simulink subsystem "Sensores_IR"  (R2023b)
settings: Solver=VariableStepAuto  StartTime=0.0  StopTime=10.0  RelTol=1e-3
libraries: arduinolib x2
settings Model: Creator=Usuario_UMA  LastModifiedBy=javie

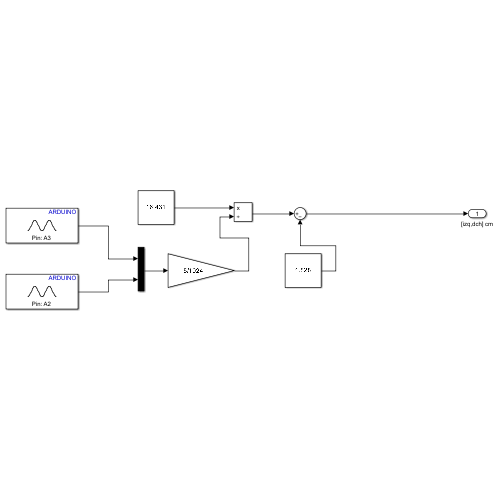
[thumbnail: Simulink's stored preview of the top-level diagram]
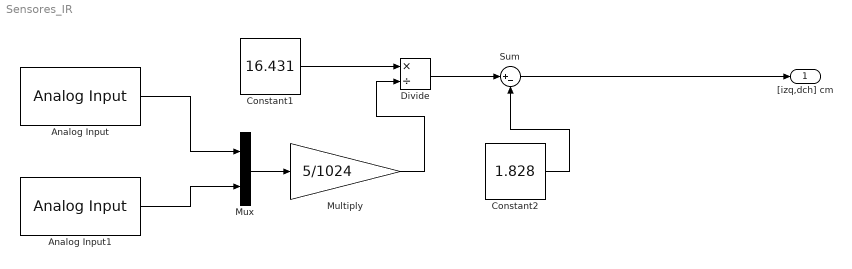
== system Sensores_IR ==
  Analog Input : arduinolib/Analog Input  pinNumber=3  ReadResultsOnly=off  ConversionTriggerSource=Software  ExternalTriggerType=uint32( 0 )  OutputDataType=uint16  EnableConversionCompleteNotify=off  EnableOuputStatus=off  SampleTime=-1  blockPlatform=arduino
  Analog Input1 : arduinolib/Analog Input  pinNumber=2  ReadResultsOnly=off  ConversionTriggerSource=Software  ExternalTriggerType=uint32( 0 )  OutputDataType=uint16  EnableConversionCompleteNotify=off  EnableOuputStatus=off  SampleTime=-1  blockPlatform=arduino
  Constant1 : Constant  Value=16.431
  Constant2 : Constant  Value=1.828
  Divide : Product  Inputs=*/
  Multiply : Gain  Gain=5/1024
  Mux : Mux  Inputs=2
  Sum : Sum  Inputs=|+-
  "[izq,dch] cm" : Outport
  wires:
  Multiply/1 -> Divide/2
  Constant1/1 -> Divide/1
  Constant2/1 -> Sum/2
  Divide/1 -> Sum/1
  Sum/1 -> "[izq,dch] cm"/1
  Mux/1 -> Multiply/1
  Analog Input/1 -> Mux/1
  Analog Input1/1 -> Mux/2
